simulink model "pt2_signal2_deadzone"  (R2019a)
settings: Solver=ode4  StartTime=0.0  StopTime=0.1  FixedStep=1e-4  RelTol=1e-3
settings Model: Creator=guima  LastModifiedBy=guima

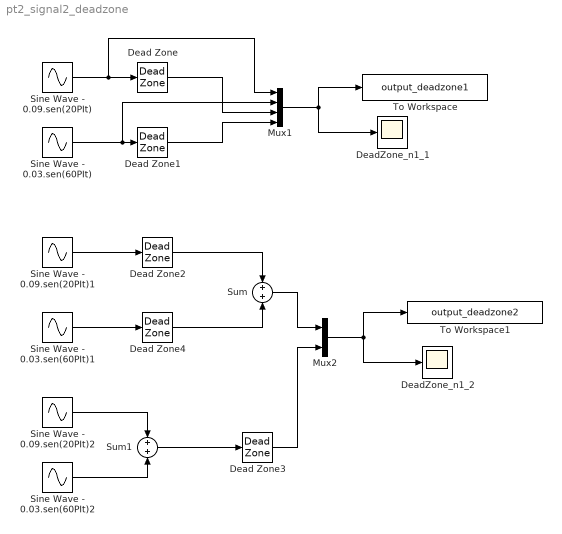
== system pt2_signal2_deadzone ==
  Dead Zone{,1..4} (5 alike) : DeadZone  LowerValue=-0.05  UpperValue=0.05  SaturateOnIntegerOverflow=on
  "DeadZone_n1_1 " : Scope
  DeadZone_n1_2 : Scope
  Mux1 : Mux
  Mux2 : Mux  Inputs=2
  Sine Wave - 0.03.sen(60PIt) : Sin  Amplitude=0.03  Frequency=60*pi  Phase=180  SampleTime=0
  Sine Wave - 0.03.sen(60PIt)1 : Sin  Amplitude=0.03  Frequency=60*pi  Phase=180  SampleTime=0
  Sine Wave - 0.03.sen(60PIt)2 : Sin  Amplitude=0.03  Frequency=60*pi  Phase=180  SampleTime=0
  Sine Wave - 0.09.sen(20PIt) : Sin  Amplitude=0.09  Frequency=20*pi  SampleTime=0
  Sine Wave - 0.09.sen(20PIt)1 : Sin  Amplitude=0.09  Frequency=20*pi  SampleTime=0
  Sine Wave - 0.09.sen(20PIt)2 : Sin  Amplitude=0.09  Frequency=20*pi  SampleTime=0
  Sum : Sum
  Sum1 : Sum
  To Workspace : ToWorkspace  VariableName=output_deadzone1  SaveFormat=Structure With Time  SampleTime=-1
  To Workspace1 : ToWorkspace  VariableName=output_deadzone2  SaveFormat=Structure With Time  SampleTime=-1
  wires:
  Mux1/1 -> "DeadZone_n1_1 "/1, To Workspace/1
  Sine Wave - 0.03.sen(60PIt)/1 -> Mux1/2, Dead Zone1/1
  Sine Wave - 0.09.sen(20PIt)/1 -> Mux1/1, Dead Zone/1
  Dead Zone/1 -> Mux1/3
  Dead Zone1/1 -> Mux1/4
  Sine Wave - 0.09.sen(20PIt)1/1 -> Dead Zone2/1
  Mux2/1 -> DeadZone_n1_2/1, To Workspace1/1
  Sine Wave - 0.03.sen(60PIt)1/1 -> Dead Zone4/1
  Dead Zone2/1 -> Sum/1
  Dead Zone4/1 -> Sum/2
  Sum/1 -> Mux2/1
  Sine Wave - 0.09.sen(20PIt)2/1 -> Sum1/1
  Sine Wave - 0.03.sen(60PIt)2/1 -> Sum1/2
  Sum1/1 -> Dead Zone3/1
  Dead Zone3/1 -> Mux2/2
